simulink model "oloop2t"  (Simulink 2.09)
settings: Solver=ode45  StartTime=0.0  StopTime=120  MaxStep=1  RelTol=1e-7  AbsTol=1e-7
undefined symbols (not defined in the file or in its folder): sfunyst, uaero0, uprop0
libraries: wndlib2 x9
settings Model: SaveTime=off  SaveOutput=off  ConsistencyChecking=off  RTWTemplateMakefile=grt_vc.tmf

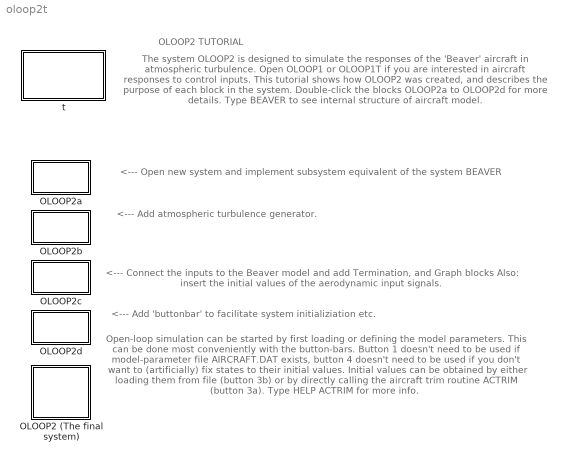
== system oloop2t ==
  note: <--- Connect the inputs to the Beaver model and add Termination, and Graph blocks
      | Also: insert the initial values of the aerodynamic  input signals.
  note: <--- Open new system and implement subsystem equivalent of the system BEAVER
  note: Open-loop simulation can be started by first loading or defining the model parameters.
      | This can be done most conveniently with the button-bars. Button 1 doesn't need to
      | be used if model-parameter file AIRCRAFT.DAT exists, button 4 doesn't need to be
      |  used if you don't want to (artificially) fix states to their initial values. Initial values can be
      | obtained by either loading them from file (button 3b) or by directly calling the aircraft
      | trim routine ACTRIM (button 3a). Type HELP ACTRIM for more info.
  note: The system OLOOP2 is designed to simulate the responses of the 'Beaver' aircraft in
      | atmospheric turbulence. Open OLOOP1 or OLOOP1T if you are interested in aircraft
      | responses to control inputs. This tutorial shows how OLOOP2 was created, and
      | describes the purpose of each block in the system. Double-click the blocks OLOOP2a
      | to OLOOP2d for more details. Type BEAVER to see internal structure of aircraft model.
  note: <--- Add atmospheric turbulence generator.
  note: <--- Add 'buttonbar' to facilitate system initializiation etc.
  note: OLOOP2 TUTORIAL
  OLOOP2 (The final system) : Subsystem
      settings: OpenFcn=oloop2
  OLOOP2a : Subsystem
  OLOOP2b : Subsystem
  OLOOP2c : Subsystem
  OLOOP2d : Subsystem
  t : Subsystem
      settings: OpenFcn=fdchelp oloop
      mask Display: disp('OLOOP2T\nMarc Rauw\nJanuary 1998')

== system oloop2t/OLOOP2 (The final system) ==

== system oloop2t/OLOOP2a ==
  note: Construction of OLOOP2
  note: Step 1: open a new system
  note: Step 2: open the main FDC library FDCLIB by typing fdclib at the Matlab command-line
  note: Step 3: double-click the upper-right, light blue block (subsystem equivalents of the model BEAVER),
      | and copy the open-loop version of these subsystems to the new Simulink system
  note: Note: here a dummy version of  this
      | model has been used to reduce the
      | file-size of the tutorial
  Beaver model : Subsystem
  wires:
  Beaver model/1(V) -> ?
  Beaver model/2(alpha) -> ?
  Beaver model/3(beta) -> ?
  Beaver model/4(p) -> ?
  Beaver model/5(q) -> ?
  Beaver model/6(r) -> ?
  Beaver model/7(psi) -> ?
  Beaver model/8(theta) -> ?
  Beaver model/9(phi) -> ?
  Beaver model/10(xe) -> ?
  Beaver model/11(ye) -> ?
  Beaver model/12(H) -> ?
  Beaver model/13(H dot) -> ?
  Beaver model/14(pb/2V) -> ?
  Beaver model/15(qc/V) -> ?
  Beaver model/16(rb/2V) -> ?
  ? -> Beaver model/1(uaero)
  ? -> Beaver model/2(uprop)
  ? -> Beaver model/3(uwind)

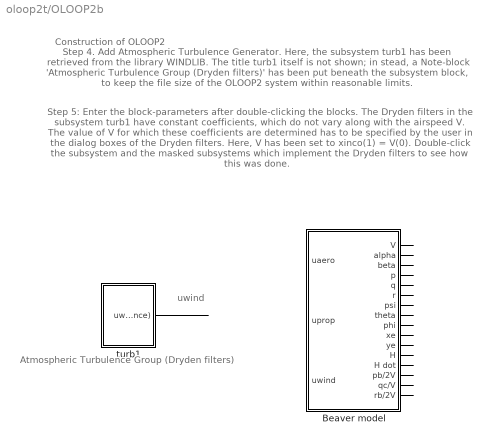
== system oloop2t/OLOOP2b ==
  note: Construction of OLOOP2
  note: Step 5: Enter the block-parameters after double-clicking the blocks. The Dryden filters in the
      | subsystem turb1 have constant coefficients, which do not vary along with the airspeed V.
      | The value of V for which these coefficients are determined has to be specified by the user in
      | the dialog boxes of the Dryden filters. Here, V has been set to  xinco(1) = V(0). Double-click
      | the subsystem and the masked subsystems which implement the Dryden filters to see how this
      | was done.
  note: Step 4. Add Atmospheric Turbulence Generator. Here, the subsystem turb1 has been retrieved
      | from the library WINDLIB. The title turb1 itself is not shown; in stead, a Note-block 'Atmospheric
      | Turbulence Group (Dryden filters)' has been put beneath the subsystem block, to keep the file
      | size of the OLOOP2 system within reasonable limits.
  note: uwind
  note: Atmospheric Turbulence
      | Group (Dryden filters)
  Beaver model : Subsystem
  turb1 : Subsystem
  wires:
  Beaver model/1(V) -> ?
  Beaver model/2(alpha) -> ?
  Beaver model/3(beta) -> ?
  Beaver model/4(p) -> ?
  Beaver model/5(q) -> ?
  Beaver model/6(r) -> ?
  Beaver model/7(psi) -> ?
  Beaver model/8(theta) -> ?
  Beaver model/9(phi) -> ?
  Beaver model/10(xe) -> ?
  Beaver model/11(ye) -> ?
  Beaver model/12(H) -> ?
  Beaver model/13(H dot) -> ?
  Beaver model/14(pb/2V) -> ?
  Beaver model/15(qc/V) -> ?
  Beaver model/16(rb/2V) -> ?
  ? -> Beaver model/1(uaero)
  ? -> Beaver model/2(uprop)
  ? -> Beaver model/3(uwind)
  turb1/1(uwind (due to turbulence)) -> ?

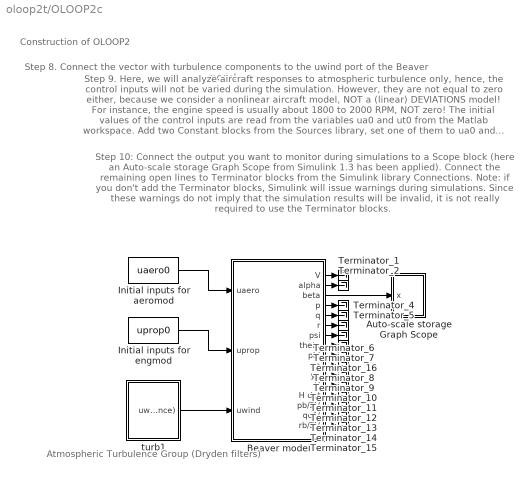
== system oloop2t/OLOOP2c ==
  note: Construction of OLOOP2
  note: Atmospheric Turbulence
      | Group (Dryden filters)
  note: Step 8. Connect the vector with turbulence components to the uwind port of the Beaver model.
  note: Step 9. Here, we will analyze aircraft responses to atmospheric turbulence only, hence, the control inputs will not be varied
      | during the simulation. However, they are not equal to zero either, because we consider a nonlinear aircraft model, NOT a
      | (linear) DEVIATIONS model! For instance, the engine speed is usually about 1800 to 2000 RPM, NOT zero! The initial values
      | of the control inputs are read from the variables ua0 and ut0 from the Matlab workspace. Add two Constant blocks from
      | the Sources library, set one of them to ua0 and the other to ut0 after double-clicking the blocks, and connect the Constant
      | blocks to the Mux block as shown in the system. We now always need to define ua0 and ut0 in the Matlab workspace!
  note: Step 10: Connect the output you want to monitor during simulations to a Scope block (here an Auto-scale storage Graph Scope
      | from Simulink 1.3 has been applied). Connect the remaining open lines to Terminator blocks from the Simulink library Connections.
      | Note: if you don't add the Terminator blocks, Simulink will issue warnings during simulations. Since these warnings do not imply
      | that the simulation results will be invalid, it is not really required  to use the Terminator blocks.
  Auto-scale storage Graph Scope : Subsystem  mask(Storage scope.){@1=5, @2=-0.02, @3=0.02, @4=200, @5='r-'}
      mask prompts: @1 "Initial Time Range:"; @2 "Initial y-min:"; @3 "Initial y-max:"; @4 "Storage pts.:"; @5 "Line type (rgbw-.:xo):"
      mask help:
      | Storage scope using MATLAB graph window.
      | Enter plotting ranges and line type.
      mask init:
      | npts = @4; color = @5; ax = [0, @1, @2, @3];
      mask Help: Uses MATLAB's graph window.\nUse only one block per system.\nLine type must be in quotes.\nSee the M-file sfunyst.m.
      mask Display: plot(0,0,100,100,[83,76,63,52,42,38,28,16,11,84,11,11,11,90,90,11],[75,58,47,54,72,80,84,74,65,65,65,90,40,40,90,90])
  Beaver model : Subsystem
  Initial inputs for aeromod : Constant  Value=uaero0
  Initial inputs for engmod : Constant  Value=uprop0
  Terminator_{1..2,4..16} (15 alike) : Terminator
  turb1 : Subsystem
  wires:
  turb1/1(uwind (due to turbulence)) -> Beaver model/3(uwind)
  Initial inputs for engmod/1 -> Beaver model/2(uprop)
  Initial inputs for aeromod/1 -> Beaver model/1(uaero)
  Beaver model/8(theta) -> Terminator_16/1
  Beaver model/2(alpha) -> Terminator_2/1
  Beaver model/3(beta) -> Auto-scale storage Graph Scope/1(x)
  Beaver model/4(p) -> Terminator_4/1
  Beaver model/5(q) -> Terminator_5/1
  Beaver model/6(r) -> Terminator_6/1
  Beaver model/7(psi) -> Terminator_7/1
  Beaver model/9(phi) -> Terminator_8/1
  Beaver model/10(xe) -> Terminator_9/1
  Beaver model/11(ye) -> Terminator_10/1
  Beaver model/12(H) -> Terminator_11/1
  Beaver model/13(H dot) -> Terminator_12/1
  Beaver model/14(pb/2V) -> Terminator_13/1
  Beaver model/15(qc/V) -> Terminator_14/1
  Beaver model/16(rb/2V) -> Terminator_15/1
  Beaver model/1(V) -> Terminator_1/1

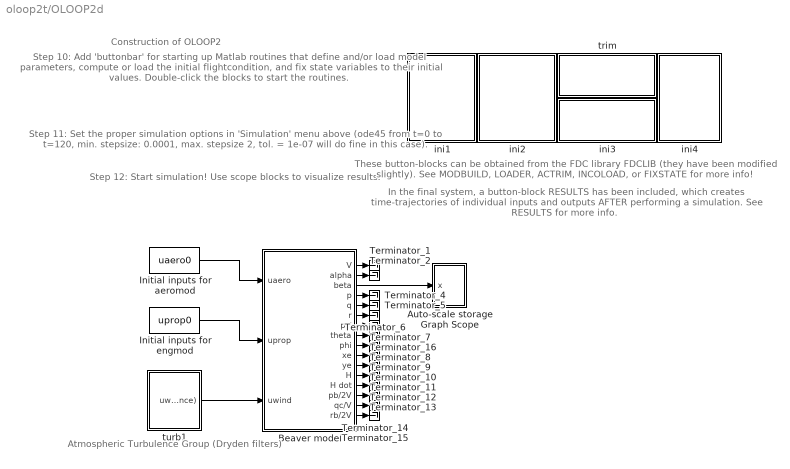
== system oloop2t/OLOOP2d ==
  note: Construction of OLOOP2
  note: In the final system, a button-block RESULTS has been included,
      | which creates time-trajectories of individual inputs and outputs
      | AFTER performing a simulation. See RESULTS for more info.
  note: Step 11: Set the proper simulation options in 'Simulation' menu
      | above (ode45 from t=0 to t=120, min. stepsize: 0.0001,
      | max. stepsize 2, tol. = 1e-07 will do fine in this case).
  note: Step 12: Start simulation! Use scope blocks to visualize results.
  note: Step 10: Add 'buttonbar' for starting up Matlab routines that
      | define and/or load model parameters, compute or load the
      | initial flightcondition, and fix state variables to their initial
      | values. Double-click the blocks to start the routines.
  note: These button-blocks can be obtained from the FDC library
      | FDCLIB (they have been modified slightly). See MODBUILD,
      | LOADER, ACTRIM, INCOLOAD, or FIXSTATE for more info!
  note: Atmospheric Turbulence
      | Group (Dryden filters)
  Auto-scale storage Graph Scope : Subsystem  mask(Storage scope.){@1=5, @2=-0.02, @3=0.02, @4=200, @5='r-'}
      mask prompts: @1 "Initial Time Range:"; @2 "Initial y-min:"; @3 "Initial y-max:"; @4 "Storage pts.:"; @5 "Line type (rgbw-.:xo):"
      mask help:
      | Storage scope using MATLAB graph window.
      | Enter plotting ranges and line type.
      mask init:
      | npts = @4; color = @5; ax = [0, @1, @2, @3];
      mask Help: Uses MATLAB's graph window.\nUse only one block per system.\nLine type must be in quotes.\nSee the M-file sfunyst.m.
      mask Display: plot(0,0,100,100,[83,76,63,52,42,38,28,16,11,84,11,11,11,90,90,11],[75,58,47,54,72,80,84,74,65,65,65,90,40,40,90,90])
  Beaver model : Subsystem
  Initial inputs for aeromod : Constant  Value=uaero0
  Initial inputs for engmod : Constant  Value=uprop0
  Terminator_{1..2,4..16} (15 alike) : Terminator
  ini1 : Subsystem
      settings: OpenFcn=modbuild
      mask Type: modbuild
      mask Display: disp('(1). Create\ndatafiles\n\n\nMODBUILD')
  ini2 : Subsystem
      settings: OpenFcn=loader
      mask Type: loader
      mask Display: disp('2. Load model\nparameters\nfrom file\n\nLOADER')
  ini3 : Subsystem
      settings: OpenFcn=incoload
      mask Type: incoload
      mask Display: disp('3b. Load initial\ncondition from file\nINCOLOAD')
  ini4 : Subsystem
      settings: OpenFcn=fixstate
      mask Type: fixstate
      mask Display: disp('(4). Fix\nindividual\nstates\n\nFIXSTATE')
  trim : Subsystem
      settings: OpenFcn=actrim
      mask Type: aircraft trim
      mask Display: disp('3a. Call aircraft\ntrim routine\nACTRIM')
  turb1 : Subsystem
  wires:
  turb1/1(uwind (due to turbulence)) -> Beaver model/3(uwind)
  Initial inputs for engmod/1 -> Beaver model/2(uprop)
  Initial inputs for aeromod/1 -> Beaver model/1(uaero)
  Beaver model/8(theta) -> Terminator_16/1
  Beaver model/2(alpha) -> Terminator_2/1
  Beaver model/3(beta) -> Auto-scale storage Graph Scope/1(x)
  Beaver model/4(p) -> Terminator_4/1
  Beaver model/5(q) -> Terminator_5/1
  Beaver model/6(r) -> Terminator_6/1
  Beaver model/7(psi) -> Terminator_7/1
  Beaver model/9(phi) -> Terminator_8/1
  Beaver model/10(xe) -> Terminator_9/1
  Beaver model/11(ye) -> Terminator_10/1
  Beaver model/12(H) -> Terminator_11/1
  Beaver model/13(H dot) -> Terminator_12/1
  Beaver model/14(pb/2V) -> Terminator_13/1
  Beaver model/15(qc/V) -> Terminator_14/1
  Beaver model/16(rb/2V) -> Terminator_15/1
  Beaver model/1(V) -> Terminator_1/1

== system oloop2t/t ==

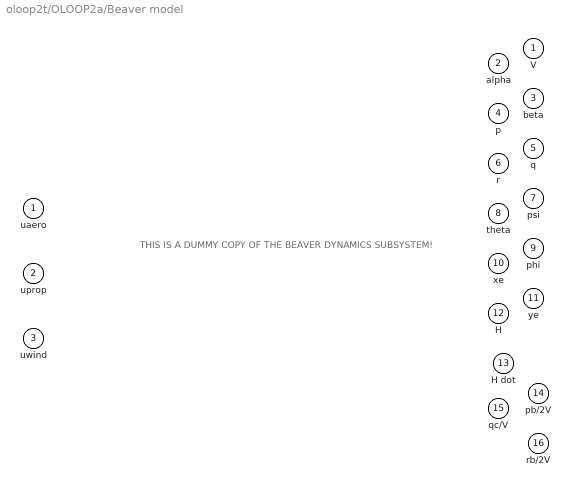
== system oloop2t/OLOOP2a/Beaver model ==
  note: THIS IS A DUMMY COPY
      | OF THE BEAVER
      | DYNAMICS SUBSYSTEM!
  uaero : Inport  Port=1  PortWidth=4  SampleTime=-1
  uprop : Inport  Port=2  PortWidth=2  SampleTime=-1
  uwind : Inport  Port=3  PortWidth=6  SampleTime=-1
  V : Outport  Port=1  InitialOutput=0
  alpha : Outport  Port=2  InitialOutput=0
  beta : Outport  Port=3  InitialOutput=0
  p : Outport  Port=4  InitialOutput=0
  q : Outport  Port=5  InitialOutput=0
  r : Outport  Port=6  InitialOutput=0
  psi : Outport  Port=7  InitialOutput=0
  theta : Outport  Port=8  InitialOutput=0
  phi : Outport  Port=9  InitialOutput=0
  xe : Outport  Port=10  InitialOutput=0
  ye : Outport  Port=11  InitialOutput=0
  H : Outport  Port=12  InitialOutput=0
  H dot : Outport  Port=13  InitialOutput=0
  pb/2V : Outport  Port=14  InitialOutput=0
  qc/V : Outport  Port=15  InitialOutput=0
  rb/2V : Outport  Port=16  InitialOutput=0

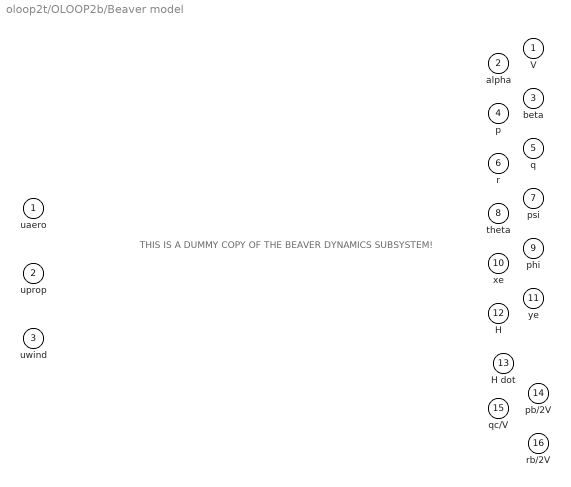
== system oloop2t/OLOOP2b/Beaver model ==
  note: THIS IS A DUMMY COPY
      | OF THE BEAVER
      | DYNAMICS SUBSYSTEM!
  uaero : Inport  Port=1  PortWidth=4  SampleTime=-1
  uprop : Inport  Port=2  PortWidth=2  SampleTime=-1
  uwind : Inport  Port=3  PortWidth=6  SampleTime=-1
  V : Outport  Port=1  InitialOutput=0
  alpha : Outport  Port=2  InitialOutput=0
  beta : Outport  Port=3  InitialOutput=0
  p : Outport  Port=4  InitialOutput=0
  q : Outport  Port=5  InitialOutput=0
  r : Outport  Port=6  InitialOutput=0
  psi : Outport  Port=7  InitialOutput=0
  theta : Outport  Port=8  InitialOutput=0
  phi : Outport  Port=9  InitialOutput=0
  xe : Outport  Port=10  InitialOutput=0
  ye : Outport  Port=11  InitialOutput=0
  H : Outport  Port=12  InitialOutput=0
  H dot : Outport  Port=13  InitialOutput=0
  pb/2V : Outport  Port=14  InitialOutput=0
  qc/V : Outport  Port=15  InitialOutput=0
  rb/2V : Outport  Port=16  InitialOutput=0

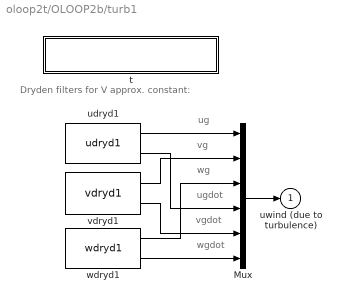
== system oloop2t/OLOOP2b/turb1 ==
  note: Dryden filters for V
      | approx. constant:
  note: ug
  note: vg
  note: wg
  note: ugdot
  note: vgdot
  note: wgdot
  Mux : Mux  Inputs=6
  t : Subsystem
      settings: OpenFcn=fdchelp turb1
      mask Display: disp('Atmospheric Turbulence Group 1\nMarc Rauw')
  "udryd1 " : wndlib2/udryd1   MaskParam1=150  MaskParam2=1  MaskParam3=45
  "vdryd1 " : wndlib2/vdryd1   MaskParam1=150  MaskParam2=1  MaskParam3=45
  "wdryd1 " : wndlib2/wdryd1   MaskParam1=150  MaskParam2=1  MaskParam3=45
  uwind (due to turbulence) : Outport  Port=1  InitialOutput=0
  wires:
  "udryd1 "/1 -> Mux/1
  "udryd1 "/2 -> Mux/4
  "wdryd1 "/2 -> Mux/6
  "wdryd1 "/1 -> Mux/3
  "vdryd1 "/2 -> Mux/5
  Mux/1 -> uwind (due to turbulence)/1
  "vdryd1 "/1 -> Mux/2

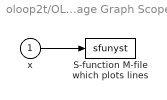
== system oloop2t/OLOOP2c/Auto-scale storage Graph Scope ==
  x : Inport  Port=1  PortWidth=-1  SampleTime=-1
  "S-function M-file which plots lines " : S-Function  LoadFcn=sfunyst([],[],[],'LoadBlock')  FunctionName=sfunyst  Parameters=ax, color, npts
      settings: CopyFcn=sfunyst([],[],[],'CopyBlock')  DeleteFcn=sfunyst([],[],[],'DeleteBlock')
  wires:
  x/1 -> "S-function M-file which plots lines "/1

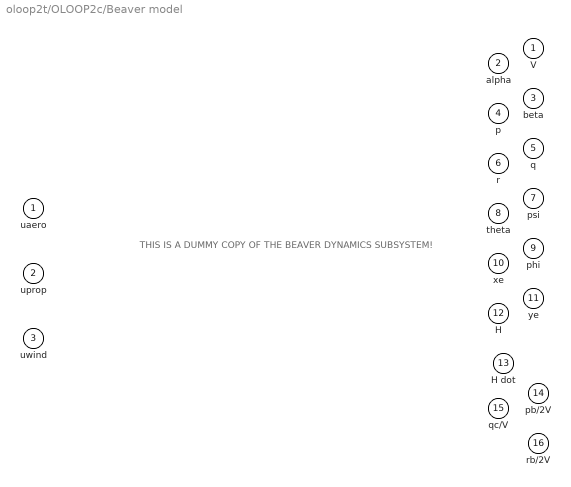
== system oloop2t/OLOOP2c/Beaver model ==
  note: THIS IS A DUMMY COPY
      | OF THE BEAVER
      | DYNAMICS SUBSYSTEM!
  uaero : Inport  Port=1  PortWidth=4  SampleTime=-1
  uprop : Inport  Port=2  PortWidth=2  SampleTime=-1
  uwind : Inport  Port=3  PortWidth=6  SampleTime=-1
  V : Outport  Port=1  InitialOutput=0
  alpha : Outport  Port=2  InitialOutput=0
  beta : Outport  Port=3  InitialOutput=0
  p : Outport  Port=4  InitialOutput=0
  q : Outport  Port=5  InitialOutput=0
  r : Outport  Port=6  InitialOutput=0
  psi : Outport  Port=7  InitialOutput=0
  theta : Outport  Port=8  InitialOutput=0
  phi : Outport  Port=9  InitialOutput=0
  xe : Outport  Port=10  InitialOutput=0
  ye : Outport  Port=11  InitialOutput=0
  H : Outport  Port=12  InitialOutput=0
  H dot : Outport  Port=13  InitialOutput=0
  pb/2V : Outport  Port=14  InitialOutput=0
  qc/V : Outport  Port=15  InitialOutput=0
  rb/2V : Outport  Port=16  InitialOutput=0

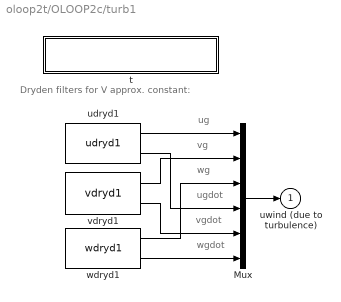
== system oloop2t/OLOOP2c/turb1 ==
  note: Dryden filters for V
      | approx. constant:
  note: ug
  note: vg
  note: wg
  note: ugdot
  note: vgdot
  note: wgdot
  Mux : Mux  Inputs=6
  t : Subsystem
      settings: OpenFcn=fdchelp turb1
      mask Display: disp('Atmospheric Turbulence Group 1\nMarc Rauw')
  "udryd1 " : wndlib2/udryd1   MaskParam1=150  MaskParam2=1  MaskParam3=45
  "vdryd1 " : wndlib2/vdryd1   MaskParam1=150  MaskParam2=1  MaskParam3=45
  "wdryd1 " : wndlib2/wdryd1   MaskParam1=150  MaskParam2=1  MaskParam3=45
  uwind (due to turbulence) : Outport  Port=1  InitialOutput=0
  wires:
  "udryd1 "/1 -> Mux/1
  "udryd1 "/2 -> Mux/4
  "wdryd1 "/2 -> Mux/6
  "wdryd1 "/1 -> Mux/3
  "vdryd1 "/2 -> Mux/5
  Mux/1 -> uwind (due to turbulence)/1
  "vdryd1 "/1 -> Mux/2

== system oloop2t/OLOOP2d/Auto-scale storage Graph Scope ==
  x : Inport  Port=1  PortWidth=-1  SampleTime=-1
  "S-function M-file which plots lines " : S-Function  LoadFcn=sfunyst([],[],[],'LoadBlock')  FunctionName=sfunyst  Parameters=ax, color, npts
      settings: CopyFcn=sfunyst([],[],[],'CopyBlock')  DeleteFcn=sfunyst([],[],[],'DeleteBlock')
  wires:
  x/1 -> "S-function M-file which plots lines "/1

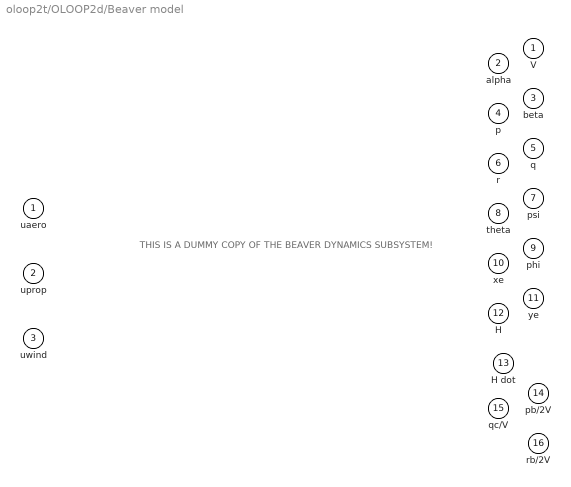
== system oloop2t/OLOOP2d/Beaver model ==
  note: THIS IS A DUMMY COPY
      | OF THE BEAVER
      | DYNAMICS SUBSYSTEM!
  uaero : Inport  Port=1  PortWidth=4  SampleTime=-1
  uprop : Inport  Port=2  PortWidth=2  SampleTime=-1
  uwind : Inport  Port=3  PortWidth=6  SampleTime=-1
  V : Outport  Port=1  InitialOutput=0
  alpha : Outport  Port=2  InitialOutput=0
  beta : Outport  Port=3  InitialOutput=0
  p : Outport  Port=4  InitialOutput=0
  q : Outport  Port=5  InitialOutput=0
  r : Outport  Port=6  InitialOutput=0
  psi : Outport  Port=7  InitialOutput=0
  theta : Outport  Port=8  InitialOutput=0
  phi : Outport  Port=9  InitialOutput=0
  xe : Outport  Port=10  InitialOutput=0
  ye : Outport  Port=11  InitialOutput=0
  H : Outport  Port=12  InitialOutput=0
  H dot : Outport  Port=13  InitialOutput=0
  pb/2V : Outport  Port=14  InitialOutput=0
  qc/V : Outport  Port=15  InitialOutput=0
  rb/2V : Outport  Port=16  InitialOutput=0

== system oloop2t/OLOOP2d/ini1 ==

== system oloop2t/OLOOP2d/ini2 ==

== system oloop2t/OLOOP2d/ini3 ==

== system oloop2t/OLOOP2d/ini4 ==

== system oloop2t/OLOOP2d/trim ==
  note: This block is used to set the initial values of the
      | state variables of the aircraft model.
      |
      | x = [V alpha beta p q r psi theta phi xe ye H]'
      |
      | x0 is stored in the file EQMINCO.mat and loaded
      | by the integrator block of the aircraft model.

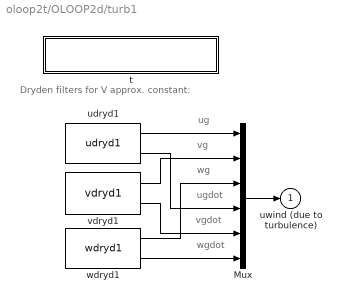
== system oloop2t/OLOOP2d/turb1 ==
  note: Dryden filters for V
      | approx. constant:
  note: ug
  note: vg
  note: wg
  note: ugdot
  note: vgdot
  note: wgdot
  Mux : Mux  Inputs=6
  t : Subsystem
      settings: OpenFcn=fdchelp turb1
      mask Display: disp('Atmospheric Turbulence Group 1\nMarc Rauw')
  "udryd1 " : wndlib2/udryd1   MaskParam1=150  MaskParam2=1  MaskParam3=45
  "vdryd1 " : wndlib2/vdryd1   MaskParam1=150  MaskParam2=1  MaskParam3=45
  "wdryd1 " : wndlib2/wdryd1   MaskParam1=150  MaskParam2=1  MaskParam3=45
  uwind (due to turbulence) : Outport  Port=1  InitialOutput=0
  wires:
  "udryd1 "/1 -> Mux/1
  "udryd1 "/2 -> Mux/4
  "wdryd1 "/2 -> Mux/6
  "wdryd1 "/1 -> Mux/3
  "vdryd1 "/2 -> Mux/5
  Mux/1 -> uwind (due to turbulence)/1
  "vdryd1 "/1 -> Mux/2

== system oloop2t/OLOOP2b/turb1/t ==

== system oloop2t/OLOOP2c/turb1/t ==

== system oloop2t/OLOOP2d/turb1/t ==
